simulink model "BD_PAR_CVT"  (Simulink 4.1.1)
settings: Solver=ode1  SolverMode=SingleTasking  StartTime=0.0  StopTime=max(cyc_mph(:,1))  FixedStep=1  MaxStep=1  RelTol=1e-3  AbsTol=1e-3
undefined symbols (not defined in the file): ess_on, ex_calc, fc_emis, fc_max_trq, fc_trq_scale, mc_max_trq, mc_overtrq_factor, mc_trq_scale, vc_idle_spd
libraries: lib_transmission x4, lib_wheel x2, lib_controls x2, lib_help x2, lib_accessory x2, lib_outputs x1, lib_interactive x1, lib_drive_cycle x1, lib_energy_storage x1, lib_exhaust x1, lib_fuel_converter x1, lib_electric_machine x1
settings Model: LastModifiedBy=ssprik  ModifiedComment=ssprik -- Wed Sep 24 15:07:48 2003 -- Version 1.22  SaveTime=off  SaveOutput=off  LimitDataPoints=off  UnconnectedLineMsg=none  RTWTemplateMakefile=grt_vc.tmf  ExtModeTrigMode=oneshot  ExtModeArmWhenConnect=off
settings Model: ModifiedHistory=|
  | ssprik -- Wed Sep 24 15:07:48 2003 -- Version 1.22
  | 
  | 
  | abrooker -- Mon Feb 10 13:02:08 2003 -- Version 1.21
  | 
  | 
  | abrooker -- Mon Feb 10 12:59:30 2003 -- Version 1.20
  | added altia block from dynamic graphics
  | 
  | mokeefe -- Fri Aug 30 07:46:52 2002 -- Version 1.19
  | Changed the input to "mechanical accessory loads <acc>/Mechanical Accessory Loads V2 <acc>" masked parameter input blocks. In R13, the function "not" no longer returns double 1 or double 0 for true and false but instead returns type logical (boolean). Thus, I am now multiplying by double 1 which causes a type conversion to double yielding the desired effect.
  | 
  | 
  | abrooker -- Tue May 14 11:46:17 2002 -- Version 1.18
  | 
  | 
  | mokeefe -- Thu Apr 18 08:02:52 2002 -- Version 1.17
  | saving the model:
  | o "without the model browser open"
  | o with only top-level screen visible
  | o and with "fit to view" enabled

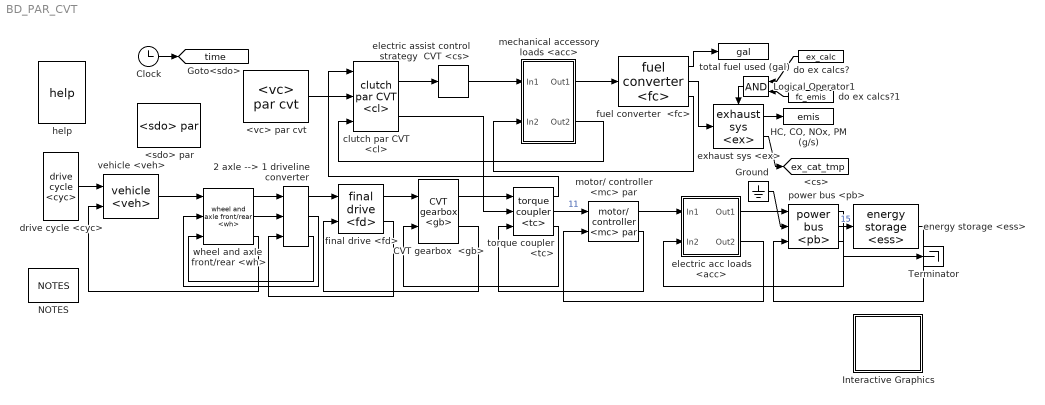
== system BD_PAR_CVT ==
  2 axle --> 1 driveline converter : lib_wheel/2 axle --> 1 driveline converter
      settings: RTWFcnNameOpts=Auto  RTWFileNameOpts=Auto
  <sdo> par : lib_outputs/<sdo> par
  <vc> par cvt : lib_controls/<vc> par cvt
      link override config traction control: BlockChoice=traction control
  CVT gearbox  <gb> : lib_transmission/CVT gearbox  <gb>
      settings: RTWFcnNameOpts=Auto  RTWFileNameOpts=Auto
  Clock : Clock
      settings: DisplayTime=off  Decimation=10
  Ground : Ground
  "HC, CO, NOx, PM (g/s)" : ToWorkspace  VariableName=emis  SampleTime=0  SaveFormat=Array
  Interactive Graphics : Subsystem  BlockChoice=on
      settings: AttributesFormatString=%<BlockChoice>  TemplateBlock=lib_interactive/Interactive Graphics  MemberBlocks=off,on  RTWFcnNameOpts=Auto  RTWFileNameOpts=Auto
  Logical Operator1 : Logic  Orientation=left  Operator=AND  Inputs=2
  NOTES : lib_help/NOTES
  Terminator : Terminator
  clutch par CVT <cl> : lib_transmission/clutch par CVT <cl>  slip_spd=vc_launch_spd  maxtrq=max(fc_max_trq)*fc_trq_scale+max(mc_max_trq)*mc_trq_scale*mc_overtrq_factor
  do ex calcs? : Constant  Orientation=left  Value=ex_calc
  do ex calcs?1 : Constant  Orientation=left  Value=fc_emis
  drive cycle <cyc> : lib_drive_cycle/drive cycle <cyc>
  electric acc loads <acc> : Subsystem
      settings: RTWFcnNameOpts=Auto  RTWFileNameOpts=Auto
      mask Display: image(imread('bdi_acc_elec.bmp'))
  electric assist control strategy  CVT <cs> : lib_controls/electric assist control strategy  CVT <cs>
  energy storage <ess> : lib_energy_storage/energy storage <ess>  AncestorBlock=lib_energy_storage/Subsystem/energy storage <ess>
      link override ess config: BlockChoice=energy storage <ess>
  exhaust sys <ex> : lib_exhaust/exhaust sys <ex>
  final drive <fd> : lib_transmission/final drive <fd>
  fuel converter  <fc> : lib_fuel_converter/fuel converter  <fc>
      link override fuel use and EO emis Configurable Subsystem: BlockChoice=fuel use and EO emis
  help : lib_help/help
  mechanical accessory loads <acc> : Subsystem
      settings: RTWFcnNameOpts=Auto  RTWFileNameOpts=Auto
      mask Display: image(imread('bdi_acc_pic.bmp'))
  motor/ controller <mc> par : lib_electric_machine/motor// controller <mc> par
  power bus <pb> : lib_power_bus/power bus <pb>
  torque coupler <tc> : lib_transmission/torque coupler <tc>
  total fuel used (gal) : ToWorkspace  VariableName=gal  SampleTime=0  SaveFormat=Array
  vehicle <veh> : lib_vehicle/vehicle <veh>
      link override record achieved force outputs/rolling resistance force: BlockChoice=force req'd to overcome rolling resistance (N)
      link override rolling resistance force: BlockChoice=force req'd to overcome rolling resistance (N)
      link override vehicle speed: BlockChoice=vehicle speed (m/s)
  wheel and axle  front/rear <wh> : lib_wheel/wheel and axle  front//rear <wh>
  tag scope: ex_cat_tmp=global, time=global
  wires:
  wheel and axle  front/rear <wh>/3 -> vehicle <veh>/2
  final drive <fd>/2 -> 2 axle --> 1 driveline converter/3
  final drive <fd>/1 -> CVT gearbox  <gb>/1
  drive cycle <cyc>/1 -> vehicle <veh>/1
  clutch par CVT <cl>/1 -> electric assist control strategy  CVT <cs>/1
  fuel converter  <fc>/2 -> exhaust sys <ex>/1
  do ex calcs?/1 -> Logical Operator1/1
  fuel converter  <fc>/1 -> total fuel used (gal)/1
  exhaust sys <ex>/1 -> "HC, CO, NOx, PM (g/s)"/1
  Logical Operator1/1 -> exhaust sys <ex>/Enable
  do ex calcs?1/1 -> Logical Operator1/2
  Clock/1 -> [time]
  CVT gearbox  <gb>/2 -> final drive <fd>/2
  torque coupler <tc>/2 -> motor/ controller <mc> par/1  "11"
  torque coupler <tc>/3 -> CVT gearbox  <gb>/2
  torque coupler <tc>/1 -> clutch par CVT <cl>/1
  clutch par CVT <cl>/2 -> torque coupler <tc>/2
  CVT gearbox  <gb>/1 -> torque coupler <tc>/1
  <vc> par cvt/1 -> clutch par CVT <cl>/2
  motor/ controller <mc> par/2 -> torque coupler <tc>/3
  Ground/1 -> power bus <pb>/2
  power bus <pb>/2 -> energy storage <ess>/1  "15"
  power bus <pb>/1 -> Terminator/1
  energy storage <ess>/1 -> power bus <pb>/3
  exhaust sys <ex>/2 -> [ex_cat_tmp]
  motor/ controller <mc> par/1 -> electric acc loads <acc>/1(In1)
  electric acc loads <acc>/1(Out1) -> power bus <pb>/1
  power bus <pb>/3 -> electric acc loads <acc>/2(In2)
  electric acc loads <acc>/2(Out2) -> motor/ controller <mc> par/2
  electric assist control strategy  CVT <cs>/1 -> mechanical accessory loads <acc>/1(In1)
  mechanical accessory loads <acc>/1(Out1) -> fuel converter  <fc>/1
  fuel converter  <fc>/3 -> mechanical accessory loads <acc>/2(In2)
  mechanical accessory loads <acc>/2(Out2) -> clutch par CVT <cl>/3
  vehicle <veh>/1 -> wheel and axle  front/rear <wh>/1
  wheel and axle  front/rear <wh>/1 -> 2 axle --> 1 driveline converter/1
  wheel and axle  front/rear <wh>/2 -> 2 axle --> 1 driveline converter/2
  2 axle --> 1 driveline converter/1 -> final drive <fd>/1
  2 axle --> 1 driveline converter/2 -> wheel and axle  front/rear <wh>/2
  2 axle --> 1 driveline converter/3 -> wheel and axle  front/rear <wh>/3

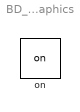
== system BD_PAR_CVT/Interactive Graphics ==
  on : lib_interactive/on  Tag=Altia_on  Orientation=up

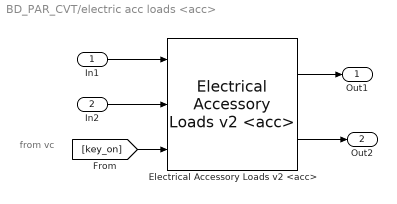
== system BD_PAR_CVT/electric acc loads <acc> ==
  note: from vc
  In1 : Inport  Port=1  LatchInput=off
  In2 : Inport  Port=2  LatchInput=off
  Electrical Accessory Loads v2 <acc> : lib_accessory/Electrical Accessory Loads v2 <acc>  load_on=ess_on
      link override backward model/electrical accessories (W): BlockChoice=Electrical Accessories: Time Variable
  Out1 : Outport  Port=1
  Out2 : Outport  Port=2
  wires:
  In1/1 -> Electrical Accessory Loads v2 <acc>/1
  In2/1 -> Electrical Accessory Loads v2 <acc>/2
  Electrical Accessory Loads v2 <acc>/1 -> Out1/1
  Electrical Accessory Loads v2 <acc>/2 -> Out2/1
  [key_on] -> Electrical Accessory Loads v2 <acc>/3

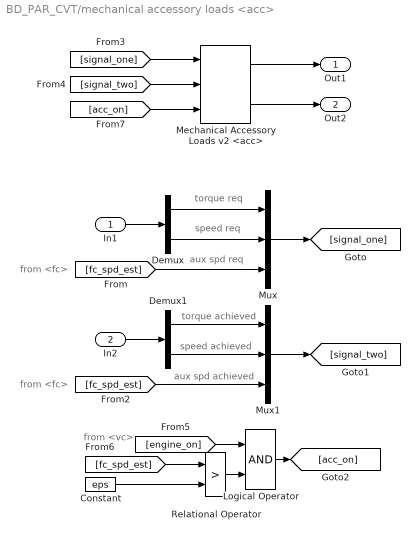
== system BD_PAR_CVT/mechanical accessory loads <acc> ==
  note: from <fc>
  note: from <fc>
  note: torque req
  note: speed req
  note: aux spd req
  note: torque achieved
  note: speed achieved
  note: aux spd achieved
  note: from <vc>
  In1 : Inport  Port=1  LatchInput=off
  In2 : Inport  Port=2  LatchInput=off
  Constant : Constant  Value=eps
  Demux : Demux  Outputs=2  BusSelectionMode=off
  Demux1 : Demux  Outputs=2  BusSelectionMode=off
  Logical Operator : Logic  Operator=AND  Inputs=2
  Mechanical Accessory Loads v2 <acc> : lib_accessory/Mechanical Accessory Loads v2 <acc>  load_on=not(ess_on)*1  acc_max_spd=inf  acc_min_spd=vc_idle_spd+eps  ic_mech_trq=0  ic_mech_pwr=0
      link override backward model/mechanical accessories (Nm): BlockChoice=Mechanical Accessories: Const Mech Var Elect
      link override estimated mechanical torque/mechanical accessories (Nm): BlockChoice=Mechanical Accessories: Const Mech Var Elect
  Mux : Mux  Inputs=3
  Mux1 : Mux  Inputs=3
  Relational Operator : RelationalOperator  Operator=>
  Out1 : Outport  Port=1
  Out2 : Outport  Port=2
  wires:
  [signal_one] -> Mechanical Accessory Loads v2 <acc>/1
  Mechanical Accessory Loads v2 <acc>/1 -> Out1/1
  Mechanical Accessory Loads v2 <acc>/2 -> Out2/1
  [signal_two] -> Mechanical Accessory Loads v2 <acc>/2
  [acc_on] -> Mechanical Accessory Loads v2 <acc>/3
  Mux/1 -> [signal_one]
  In1/1 -> Demux/1
  Demux/1 -> Mux/1
  Demux/2 -> Mux/2
  [fc_spd_est] -> Mux/3
  Mux1/1 -> [signal_two]
  In2/1 -> Demux1/1
  Demux1/1 -> Mux1/1
  Demux1/2 -> Mux1/2
  [fc_spd_est] -> Mux1/3
  [fc_spd_est] -> Relational Operator/1
  Constant/1 -> Relational Operator/2
  [engine_on] -> Logical Operator/1
  Relational Operator/1 -> Logical Operator/2
  Logical Operator/1 -> [acc_on]
